simulink library "calculateCYorCLorCN_ul"  (R2020a)
settings: Solver=VariableStepAuto  StartTime=0.0  StopTime=10.0  RelTol=1e-3
undefined symbols (not defined in the file): coeffvals
libraries: calcAeroCoeffFromPolynomial_ul x5
settings Model: Creator=Ayaz  LastModifiedBy=Ayaz

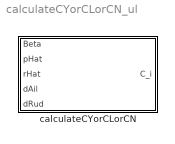
== system calculateCYorCLorCN_ul ==
  calculateCYorCLorCN : Subsystem  mask{C_i_Beta_coeffs=coeffvals, C_i_pHat_coeffs=coeffvals, C_i_rHat_coeffs=coeffvals, C_i_dAil_coeffs=coeffvals, C_i_dRud_coeffs=coeffvals}
      mask prompts: C_i_Beta_coeffs "C_i_Beta polynomial coefficients (c0,c1,c2):"; C_i_pHat_coeffs "C_i_pHat polynomial coefficients (c0,c1,c2):"; C_i_rHat_coeffs "C_i_rHat polynomial coefficients (c0,c1,c2):"; C_i_dAil_coeffs "C_i_dAil polynomial coefficients (c0,c1,c2):"; C_i_dRud_coeffs "C_i_dRud polynomial coefficients (c0,c1,c2):"
      mask TypeOptions C_i_Beta_coeffs: C_i_Beta/coeffVals
      mask TypeOptions C_i_pHat_coeffs: C_i_pHat/coeffVals
      mask TypeOptions C_i_rHat_coeffs: C_i_rHat/coeffVals
      mask TypeOptions C_i_dAil_coeffs: C_i_dAil/coeffVals
      mask TypeOptions C_i_dRud_coeffs: C_i_dRud/coeffVals

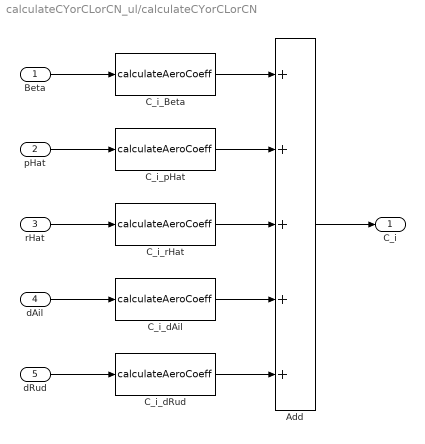
== system calculateCYorCLorCN_ul/calculateCYorCLorCN ==
  Beta : Inport
  pHat : Inport  Port=2
  rHat : Inport  Port=3
  dAil : Inport  Port=4
  dRud : Inport  Port=5
  Add : Sum  Inputs=+++++
  C_i_Beta : calcAeroCoeffFromPolynomial_ul/calculateAeroCoeff  coeffVals=C_i_Beta_coeffs
  C_i_dAil : calcAeroCoeffFromPolynomial_ul/calculateAeroCoeff  coeffVals=C_i_dAil_coeffs
  C_i_dRud : calcAeroCoeffFromPolynomial_ul/calculateAeroCoeff  coeffVals=C_i_dRud_coeffs
  C_i_pHat : calcAeroCoeffFromPolynomial_ul/calculateAeroCoeff  coeffVals=C_i_pHat_coeffs
  C_i_rHat : calcAeroCoeffFromPolynomial_ul/calculateAeroCoeff  coeffVals=C_i_rHat_coeffs
  C_i : Outport
  wires:
  Beta/1 -> C_i_Beta/1
  pHat/1 -> C_i_pHat/1
  rHat/1 -> C_i_rHat/1
  dAil/1 -> C_i_dAil/1
  dRud/1 -> C_i_dRud/1
  C_i_dRud/1 -> Add/5
  C_i_dAil/1 -> Add/4
  C_i_rHat/1 -> Add/3
  C_i_pHat/1 -> Add/2
  C_i_Beta/1 -> Add/1
  Add/1 -> C_i/1
